simulink model "untitled"  (R2012b)
settings: Solver=ode45  StartTime=0.0  StopTime=1  RelTol=1e-3
undefined symbols (not defined in the file or in its folder): jet
libraries: visionsources x2, visionsinks x2, visiongeotforms x1
settings Model: Creator=hp  LastModifiedBy=hp

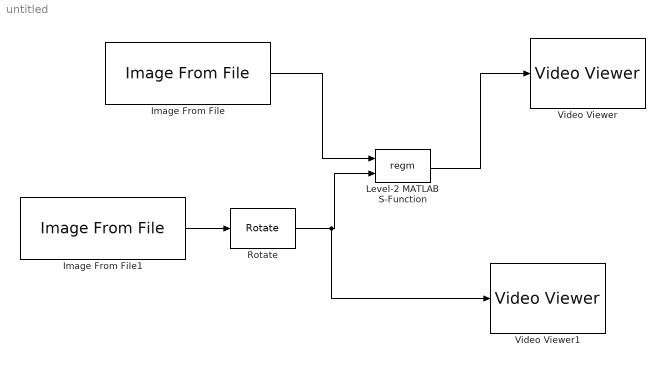
== system untitled ==
  Image From File : visionsources/Image From File  Tag=vipblks_nd  FileName=cameraman.tif  imagePorts=One multidimensional signal  Ts=inf  ImageDataType=double  Signed=on  WordLength=16  sdImageDataType=uint(8)  FractionLengthMode=User-defined  FractionLength=15  OutPortLabels=R|G|B
  Image From File1 : visionsources/Image From File  Tag=vipblks_nd  FileName=cameraman.tif  imagePorts=One multidimensional signal  Ts=inf  ImageDataType=double  Signed=on  WordLength=16  sdImageDataType=uint(8)  FractionLengthMode=User-defined  FractionLength=15  OutPortLabels=R|G|B
  Level-2 MATLAB S-Function : M-S-Function  FunctionName=regm
  Rotate : visiongeotforms/Rotate  outSizeR=Same as input image  src_angle=Specify via dialog  unit_angle=Degrees  angle=pi/2  maxAngle=pi  dispImage=Center  method=Table lookup  fillVal=0  interpMethod=Bilinear  prodOutputMode=Binary point scaling  prodOutputWordLength=32  prodOutputFracLength=10  roundingMode=Nearest  overflowMode=on
  Video Viewer : visionsinks/Video Viewer  inputType=Obsolete7b  imagePorts=One multidimensional signal  useColorMap=off  colormapValue=jet(256)  specRange=off  minInputVal=0  maxInputVal=255  FigPos=[948 591 410 300]  AxisZoom=on  trueSizedOnce=off  OpenAtMdlStart=on  DefaultConfigurationName=vipscopes.VideoViewerScopeCfg
  Video Viewer1 : visionsinks/Video Viewer  inputType=Obsolete7b  imagePorts=One multidimensional signal  useColorMap=off  colormapValue=jet(256)  specRange=off  minInputVal=0  maxInputVal=255  FigPos=[478 533 410 300]  AxisZoom=on  trueSizedOnce=off  OpenAtMdlStart=on  DefaultConfigurationName=vipscopes.VideoViewerScopeCfg
  wires:
  Image From File/1 -> Level-2 MATLAB S-Function/1
  Level-2 MATLAB S-Function/1 -> Video Viewer/1
  Rotate/1 -> Video Viewer1/1, Level-2 MATLAB S-Function/2
  Image From File1/1 -> Rotate/1
